simulink model "Simulation_Test"  (R2018a)
settings: Solver=VariableStepAuto  StartTime=0.0  StopTime=700  RelTol=1e-3
undefined symbols (not defined in the file or in its folder): sigbuilder_block
libraries: Vehicule x1
settings Model: Creator=Thomas  LastModifiedBy=thomas.moser
settings SolverCC: ZeroCrossAlgorithm=Adaptive
settings DebuggingCC: MaxConsecutiveZCsMsg=none

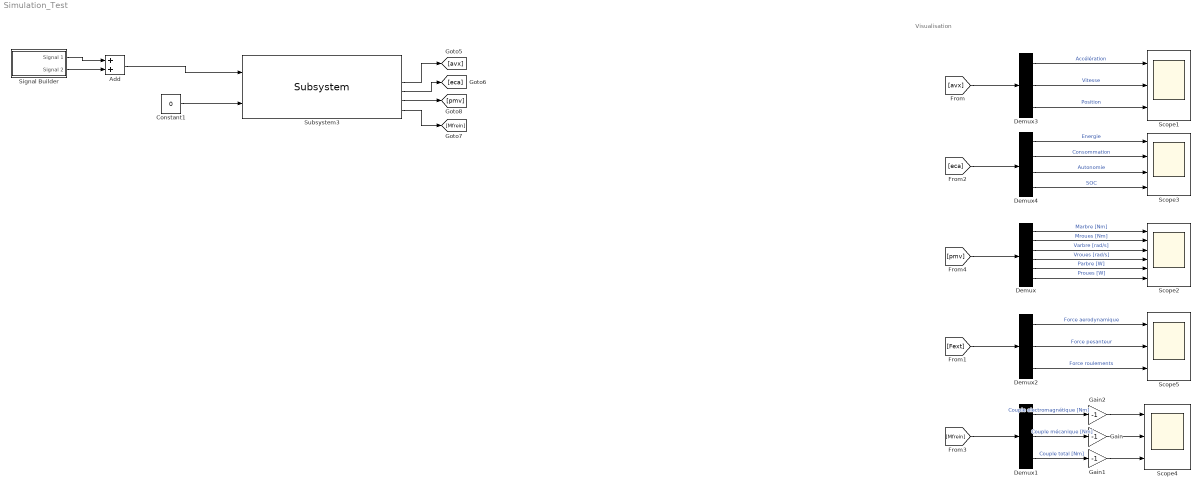
== system Simulation_Test ==
  note: Visualisation
  Add : Sum
  Constant1 : Constant  Value=0
  Demux : Demux  Outputs=6
  Demux1 : Demux  Outputs=3
  Demux2 : Demux  Outputs=3
  Demux3 : Demux  Outputs=3
  Demux4 : Demux
  Gain : Gain  Gain=-1
  Gain1 : Gain  Gain=-1
  Gain2 : Gain  Gain=-1
  Scope1 : Scope  NumInputPorts=3
  Scope2 : Scope  NumInputPorts=6
  Scope3 : Scope  NumInputPorts=4
  Scope4 : Scope  NumInputPorts=3
  Scope5 : Scope  NumInputPorts=3
  Signal Builder : Subsystem  Tag=STV Subsys  LoadFcn=sigbuilder_block('load');  StartFcn=sigbuilder_block('start');  StopFcn=sigbuilder_block('stop');  ClipboardFcn=sigbuilder_block('clipboard');  mask(Sigbuilder block){tuvar=[0:10]}
      mask help: Simulink:masks:SigbuilderBlock_MD
      mask init:
      | if ~strcmp(get_param(bdroot(gcbh),'SimulationStatus'),'stopped') tuvar = sigbuilder_block('maskInit'); end
      settings: CopyFcn=sigbuilder_block('copy');  DeleteFcn=sigbuilder_block('delete');  ModelCloseFcn=sigbuilder_block('modelClose');  PreSaveFcn=sigbuilder_block('preSave');  PauseFcn=sigbuilder_block('pause');  ContinueFcn=sigbuilder_block('continue');  NameChangeFcn=sigbuilder_block('namechange');  OpenFcn=sigbuilder_block('open',[437.6 199.2 550.4 400 ]);  CloseFcn=sigbuilder_block('close');
      mask Display: plot(0, 0, 100, 100,[2, 2, 32, 32, 2], [68, 8, 8, 68, 68],[32, 2], [38, 38], [32, 19, 2],[53, 60, 44], [32, 17, 17, 2],[16, 16, 31, 31]);txt = getActiveGroup(gcbh);text(2, 100, txt,'verticalAlignment', 'top');
  Subsystem3 : Vehicule/Subsystem  m=2250  mp=80  rr=0.33  s=1  cx=0.5  crr=0.015  mlimit=660  alimit=3  vMin=25/3.6  vMax=250/3.6  r=9.73  nr=0.9  nm=0.89  Pmin=-310380  Mmin=-660  nc=0.89  cb=98  soc=100  tempExt=25  nbrCycle=0
  wires:
  Demux/1 -> Scope2/1  "Marbre [Nm]"
  Demux/2 -> Scope2/2  "Mroues [Nm]"
  Demux/3 -> Scope2/3  "Varbre [rad/s]"
  Demux/4 -> Scope2/4  "Vroues [rad/s]"
  Demux/5 -> Scope2/5  "Parbre [W]"
  Demux/6 -> Scope2/6  "Proues [W]"
  Demux1/1 -> Gain2/1  "Couple electromagnétique [Nm]"
  Demux1/2 -> Gain/1  "Couple mécanique [Nm]"
  Demux1/3 -> Gain1/1  "Couple total [Nm]"
  [avx] -> Demux3/1
  Demux3/1 -> Scope1/1  "Accélération"
  Demux3/2 -> Scope1/2  "Vitesse"
  Demux3/3 -> Scope1/3  "Position"
  Demux2/1 -> Scope5/1  "Force aerodynamique"
  Demux2/2 -> Scope5/2  "Force pesanteur"
  Demux2/3 -> Scope5/3  "Force roulements"
  [Fext] -> Demux2/1
  Demux4/3 -> Scope3/3  "Autonomie"
  [eca] -> Demux4/1
  Demux4/1 -> Scope3/1  "Energie"
  Demux4/2 -> Scope3/2  "Consommation"
  Demux4/4 -> Scope3/4  "SOC"
  [Mfrein] -> Demux1/1
  [pmv] -> Demux/1
  Gain/1 -> Scope4/2
  Gain2/1 -> Scope4/1
  Gain1/1 -> Scope4/3
  Constant1/1 -> Subsystem3/2
  Subsystem3/3 -> [avx]
  Subsystem3/4 -> [eca]
  Subsystem3/5 -> [pmv]
  Subsystem3/6 -> [Mfrein]
  Signal Builder/1(Signal 1) -> Add/1
  Signal Builder/2(Signal 2) -> Add/2
  Add/1 -> Subsystem3/1

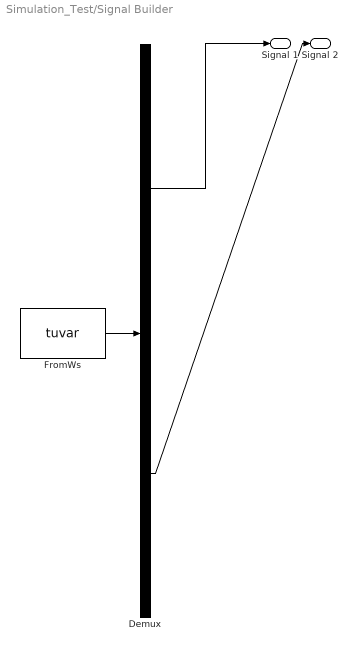
== system Simulation_Test/Signal Builder ==
  Demux : Demux  Tag=STV Demux  Outputs=2
  FromWs : FromWorkspace  Tag=STV FromWs  VariableName=tuvar  SampleTime=0
      SigBuilderData=|
      | common.afterFinalStr = 'Extrapolate'
      | common.sampleTime = 0
      | dataSet.timeRange = [0 100]
      | dataSet.name = 'Group 1'
      | sbobj.Groups.Name = 'Group 1'
      | sbobj.Groups.Signals(1).Name = 'Signal 1'
      | sbobj.Groups.Signals(1).XData = [0 20 20 100]
      | sbobj.Groups.Signals(1).YData = [660 660 0 0]
      | sbobj.Groups.Signals(2).Name = 'Signal 2'
      | sbobj.Groups.Signals(2).XData = [0 30 35 100]
      | sbobj.Groups.Signals(2).YData = [0 0 -230 -230]
      | sbobj.Groups.TimeRange = [0 100]
  Signal 1 : Outport  Tag=STV Outport
  Signal 2 : Outport  Tag=STV Outport  Port=2
  wires:
  Demux/1 -> Signal 1/1
  FromWs/1 -> Demux/1
  Demux/2 -> Signal 2/1
